simulink model "ball_on_beam_sim_HW_06"  (R2018a)
settings: Solver=ode45  StartTime=0.0  StopTime=100  MaxStep=1  RelTol=1e-3
InitFcn:
  | ball_on_beam_param
undefined symbols (not defined in the file or in its folder): ball_on_beam_animation, ball_on_beam_ctrl, Par
settings Model: Creator=canla  LastModifiedBy=canla
settings OptimizationCC: LifeSpan=inf

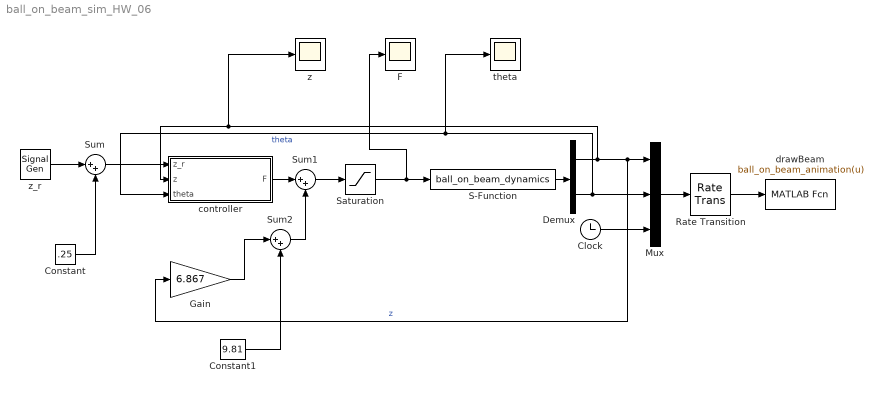
== system ball_on_beam_sim_HW_06 ==
  Clock : Clock
  Constant : Constant  Value=.25
  Constant1 : Constant  Value=9.81
  Demux : Demux  Outputs=2
  F : Scope
  Gain : Gain  Gain=6.867
  Mux : Mux  Inputs=3
  Rate Transition : RateTransition  OutPortSampleTime=Par.t_plot
  S-Function : S-Function  FunctionName=ball_on_beam_dynamics  Parameters=Par  SFunctionDeploymentMode=off  EnableBusSupport=off
  Saturation : Saturate  UpperLimit=Par.F_max  LowerLimit=-Par.F_max
  Sum : Sum  Inputs=|++
  Sum1 : Sum  Inputs=|++
  Sum2 : Sum  Inputs=|++
  controller : Subsystem
  drawBeam : MATLABFcn  MATLABFcn=ball_on_beam_animation(u)  OutputDimensions=0
  theta : Scope
  z : Scope
  z_r : SignalGenerator  WaveForm=square  Amplitude=0.15  Frequency=0.01
  wires:
  S-Function/1 -> Demux/1
  Demux/2 -> theta/1, controller/3(theta), Mux/2  "theta"
  Demux/1 -> z/1, controller/2(z), Gain/1, Mux/1  "z"
  Clock/1 -> Mux/3
  Mux/1 -> Rate Transition/1
  Rate Transition/1 -> drawBeam/1
  Gain/1 -> Sum2/1
  Saturation/1 -> F/1, S-Function/1
  controller/1(F) -> Sum1/1
  Sum2/1 -> Sum1/2
  Constant1/1 -> Sum2/2
  Sum1/1 -> Saturation/1
  Sum/1 -> controller/1(z_r)
  z_r/1 -> Sum/1
  Constant/1 -> Sum/2

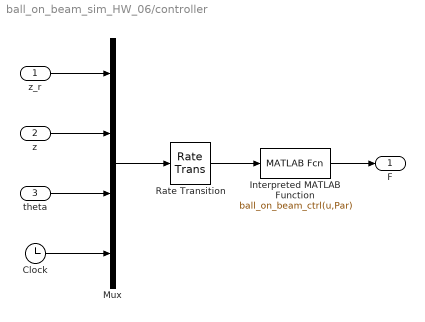
== system ball_on_beam_sim_HW_06/controller ==
  z_r : Inport
  z : Inport  Port=2
  theta : Inport  Port=3
  Clock : Clock
  Interpreted MATLAB Function : MATLABFcn  MATLABFcn=ball_on_beam_ctrl(u,Par)  OutputDimensions=1
  Mux : Mux
  Rate Transition : RateTransition  OutPortSampleTime=Par.Ts
  F : Outport
  wires:
  z/1 -> Mux/2
  z_r/1 -> Mux/1
  theta/1 -> Mux/3
  Clock/1 -> Mux/4
  Mux/1 -> Rate Transition/1
  Rate Transition/1 -> Interpreted MATLAB Function/1
  Interpreted MATLAB Function/1 -> F/1
